simulink model "GCS"  (R2024a)
settings: Solver=VariableStepAuto  StartTime=0.0  StopTime=inf  RelTol=1e-3
(part 1 of 2)
settings Model: Creator=gurt1  LastModifiedBy=gurt1

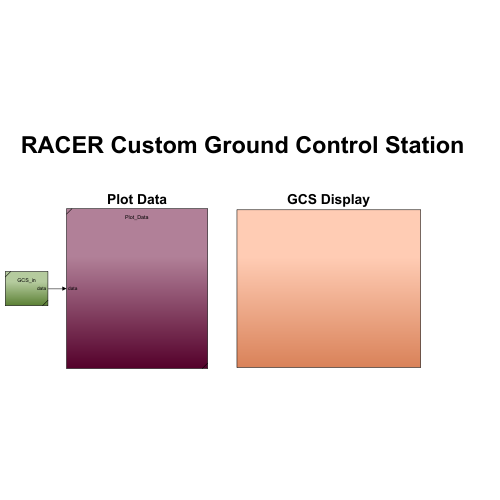
[thumbnail: Simulink's stored preview of the top-level diagram]
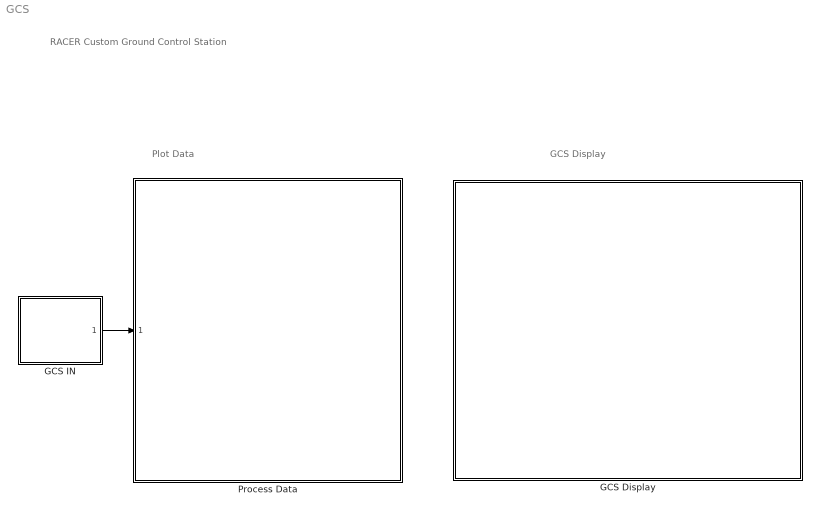
== system GCS ==
  note: Plot Data
  note: GCS Display
  note: RACER Custom Ground Control Station
  GCS Display : Subsystem
  GCS IN : Subsystem  ReferencedSubsystem=GCS_in
  Process Data : Subsystem  ReferencedSubsystem=Plot_Data
  wires:
  GCS IN/1 -> Process Data/1
